simulink model "trajectory_control_of_non_linear_flexible_arm_simulation"  (R2013a)
settings: Solver=ode45  StartTime=0.0  StopTime=10.0  RelTol=1e-3
PreLoadFcn:
  | trajectory_control_of_non_linear_flexible_arm
values from neighbouring files (symbols this model uses):
  I0 = 1    [M.m]    (also in nxxf.m; trajectory_control_of_non_linear_flexible_arm.m)
  J0 = 0.109    [M.m]    (also in nxxf.m; trajectory_control_of_non_linear_flexible_arm.m)
  Jp = 0.00852    [M.m]    (also in nxxf.m; trajectory_control_of_non_linear_flexible_arm.m)
  l = 4    [M.m]    (also in nxxf.m; trajectory_control_of_non_linear_flexible_arm.m)
  ML = 0.0031    [M.m]    (also in nxxf.m; trajectory_control_of_non_linear_flexible_arm.m)
settings Model: Creator=CUHK-RAIL-LAB  LastModifiedBy=CUHK-RAIL-LAB

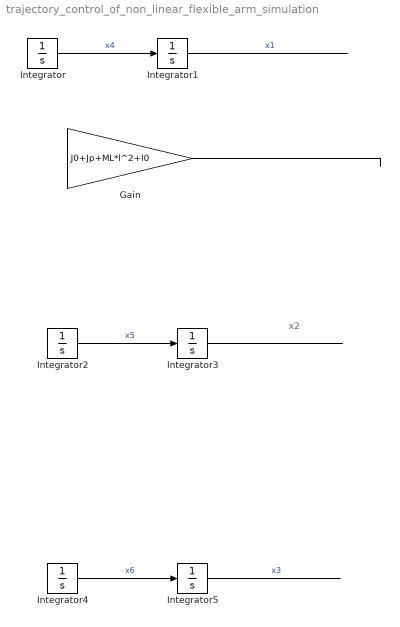
== system trajectory_control_of_non_linear_flexible_arm_simulation ==
  note: x2
  Gain : Gain  Gain=J0+Jp+ML*l^2+I0
  Integrator{,1..5} (6 alike) : Integrator
  wires:
  Integrator/1 -> Integrator1/1  "x4"
  Integrator1/1 -> ?  "x1"
  Integrator2/1 -> Integrator3/1  "x5"
  Integrator3/1 -> ?
  Integrator4/1 -> Integrator5/1  "x6"
  Integrator5/1 -> ?  "x3"
  ? -> Gain/1, Integrator/1
  ? -> Integrator2/1
  ? -> Integrator4/1
  Gain/1 -> ?
